simulink model "furuta_pendulum_v_1"  (R2018b)
settings: Solver=FixedStepAuto  StartTime=0.0  StopTime=200  FixedStep=0.001  RelTol=1e-3
settings Model: Creator=root  LastModifiedBy=root

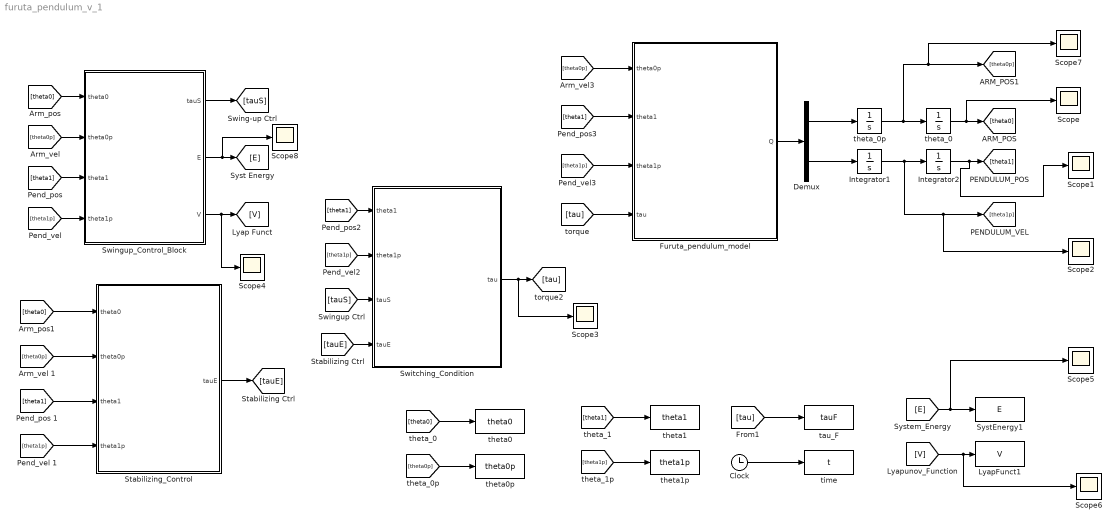
== system furuta_pendulum_v_1 ==
  Clock : Clock
  Demux : Demux  Outputs=2
  Furuta_pendulum_model : MATLAB Function  TreatAsAtomicUnit=on
  Integrator1 : Integrator
  Integrator2 : Integrator  InitialCondition=1
  LyapFunct1 : ToWorkspace  VariableName=V  SampleTime=-1
  Scope{,1..8} (9 alike) : Scope
  Stabilizing_Control : MATLAB Function  TreatAsAtomicUnit=on
  Swingup_Control_Block : MATLAB Function  TreatAsAtomicUnit=on
  Switching_Condition : MATLAB Function  TreatAsAtomicUnit=on
  SystEnergy1 : ToWorkspace  VariableName=E  SampleTime=-1
  tau_F : ToWorkspace  VariableName=tauF  SampleTime=-1
  theta0 : ToWorkspace  VariableName=theta0  SampleTime=-1
  theta0p : ToWorkspace  VariableName=theta0p  SampleTime=-1
  theta1 : ToWorkspace  VariableName=theta1  SampleTime=-1
  "theta1p " : ToWorkspace  VariableName=theta1p  SampleTime=-1
  "theta_0 " : Integrator
  theta_0p : Integrator
  time : ToWorkspace  VariableName=t  SampleTime=-1
  wires:
  Swingup_Control_Block/3(V) -> Scope4/1, [V]
  Swingup_Control_Block/2(E) -> Scope8/1, [E]
  Swingup_Control_Block/1(tauS) -> [tauS]
  [theta0] -> Swingup_Control_Block/1(theta0)
  [theta0p] -> Swingup_Control_Block/2(theta0p)
  [theta1] -> Swingup_Control_Block/3(theta1)
  [theta1p] -> Swingup_Control_Block/4(theta1p)
  [theta0] -> Stabilizing_Control/1(theta0)
  [theta0p] -> Stabilizing_Control/2(theta0p)
  [theta1] -> Stabilizing_Control/3(theta1)
  [theta1p] -> Stabilizing_Control/4(theta1p)
  Stabilizing_Control/1(tauE) -> [tauE]
  [theta1] -> Switching_Condition/1(theta1)
  [theta1p] -> Switching_Condition/2(theta1p)
  [tauS] -> Switching_Condition/3(tauS)
  [tauE] -> Switching_Condition/4(tauE)
  Switching_Condition/1(tau) -> Scope3/1, [tau]
  [theta0p] -> Furuta_pendulum_model/1(theta0p)
  [theta1] -> Furuta_pendulum_model/2(theta1)
  [theta1p] -> Furuta_pendulum_model/3(theta1p)
  [tau] -> Furuta_pendulum_model/4(tau)
  Furuta_pendulum_model/1(Q) -> Demux/1
  Demux/1 -> theta_0p/1
  theta_0p/1 -> Scope7/1, [theta0p], "theta_0 "/1
  Demux/2 -> Integrator1/1
  Integrator1/1 -> Scope2/1, [theta1p], Integrator2/1
  "theta_0 "/1 -> Scope/1, [theta0]
  Integrator2/1 -> Scope1/1, [theta1]
  [theta1] -> theta1/1
  [theta1p] -> "theta1p "/1
  [tau] -> tau_F/1
  Clock/1 -> time/1
  [V] -> Scope6/1, LyapFunct1/1
  [E] -> Scope5/1, SystEnergy1/1
  [theta0p] -> theta0p/1
  [theta0] -> theta0/1

== matlab function furuta_pendulum_v_1/Swingup_Control_Block ==
  data: theta0 input; tauS output; theta0p input; theta1 input; theta1p input; E output; V output

function [tauS,E,V] = fcn(theta0,theta0p,theta1,theta1p)

%%-------------Parameters
g = 9.81;
lpc = 129e-3;
lb = 155e-3;
mp = 22.18e-3;
J1 = 184.5e-6;
I0 = 238.49e-6;
ke = 1900;
kw =1;
kdelta = 3;
ktheta = 3;

qp=[theta0p;theta1p];
M11= I0 + mp*(lb^2) + (lpc^2)*mp*(sin(theta1)^2);
M12= mp*lb*lpc*cos(theta1);
M21= mp*lb*lpc*cos(theta1);
M22= J1 + mp*(lpc^2);
Dq=[M11 M12;
M21 M22];

detD=det(Dq);

E= (0.5)*qp'*Dq*qp + mp*g*lpc*(cos(theta1)-1);

F= -(J1 + mp*(lpc^2))*mp*(lpc^2)*sin(2*theta1)*theta0p*theta1p-... 
    (0.5)*(mp^2)*(lpc^3)*lb*cos(theta1)*sin(2*theta1)*(theta0p^2)+... 
    (J1 + mp*(lpc^2))*mp*lpc*lb*sin(theta1)*(theta1p^2)-... 
    (mp^2)*(lpc^2)*lb*g*cos(theta1)*sin(theta1);


tauS= (-kw*F-detD*(kdelta*theta0p + ktheta*theta0))...
/(detD*ke*E + kw*(J1 + mp*(lpc^2)));


V = 0.5*ke*E^2 + 0.5*kw*theta0p^2 + 0.5*ktheta*theta0^2;

== matlab function furuta_pendulum_v_1/Furuta_pendulum_model ==
  data: theta0p input; Q output; theta1 input; theta1p input; tau input
function Q = modelo(theta0p,theta1,theta1p,tau)


%%-----------Parameters-----------%%
g = 9.81;
l1 = 129e-3;
L0 = 155e-3;
m1 = 22.18e-3;
J1 = 184.5e-6;
I0 = 238.49e-6;
%%----- M(q)qpp + C(q, qp)qp + G(q) = T----%%
%%----- q=[theta0;theta1]-----------%%
M11= I0 + m1*(L0^2) + (l1^2)*m1*(sin(theta1)^2);
M12= m1*L0*l1*cos(theta1);
M21= m1*L0*l1*cos(theta1);
M22= J1 + m1*(l1^2);
M= [M11 M12;
M21 M22];
C11= 2*(l1^2)*m1*sin(theta1)*cos(theta1)*theta1p;
C12= -m1*L0*l1*sin(theta1)*theta1p;
C21= -m1*(l1^2)*sin(theta1)*cos(theta1)*theta0p;
C22= 0;
C= [C11 C12;
C21 C22];
G11= 0;
G21= -m1*g*l1*sin(theta1);
G= [G11;
G21];
T= [tau;
0];

Qp= [theta0p;
theta1p];
Qpp= M \ ( T - C*Qp - G );
theta0pp=Qpp(1,1);
theta1pp=Qpp(2,1);
Q=[theta0pp;theta1pp];

== matlab function furuta_pendulum_v_1/Stabilizing_Control ==
  data: theta0 input; tauE output; theta0p input; theta1 input; theta1p input
function tauE = fcn(theta0,theta0p,theta1,theta1p)
if(theta1>pi)
theta1d=2*pi;
else
theta1d=0;
end
x=[theta0 theta0p (theta1-theta1d) theta1p];
K=[-0.0118 -0.0118 -0.2742 -0.0298];
%K= [-0.0804 -0.0804 -0.8269 -0.1304];
tauE = -K*x';

%------------

== matlab function furuta_pendulum_v_1/Switching_Condition ==
  data: theta1 input; tau output; theta1p input; tauS input; tauE input
function tau = fcn(theta1,theta1p,tauS,tauE)

if(theta1>pi)
theta1d=2*pi;
else
theta1d=0;
end

if sqrt(3*(theta1-theta1d)^2+0.1*(theta1p*theta1p)) < 0.2
tau = tauE;
else
tau= tauS;
end
